simulink model "Type1_c"  (R2019a)
settings: Solver=VariableStepAuto  StartTime=0.0  StopTime=10.0  RelTol=1e-3
libraries: simulink x3
settings Model: Creator=admin  LastModifiedBy=admin

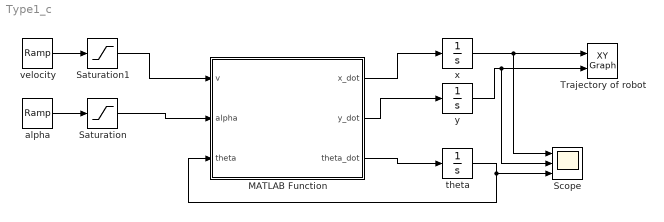
== system Type1_c ==
  MATLAB Function : MATLAB Function  TreatAsAtomicUnit=on
  Saturation : Saturate  UpperLimit=pi/4  LowerLimit=-pi/4
  Saturation1 : Saturate  UpperLimit=1.68  LowerLimit=-1.68  LinearizeAsGain=off
  Scope : Scope  NumInputPorts=3
  Trajectory of robot : simulink/Sinks/XY Graph  xmin=-2  xmax=7  ymin=-1  ymax=5  st=-1
  alpha : simulink/Sources/Ramp  slope=0.6  start=0  InitialOutput=0
  theta : Integrator
  velocity : simulink/Sources/Ramp  slope=0.3  start=0  InitialOutput=0
  x : Integrator
  y : Integrator
  wires:
  x/1 -> Trajectory of robot/1, Scope/1
  theta/1 -> Scope/3, MATLAB Function/3(theta)
  MATLAB Function/2(y_dot) -> y/1
  MATLAB Function/3(theta_dot) -> theta/1
  MATLAB Function/1(x_dot) -> x/1
  y/1 -> Scope/2, Trajectory of robot/2
  Saturation/1 -> MATLAB Function/2(alpha)
  velocity/1 -> Saturation1/1
  Saturation1/1 -> MATLAB Function/1(v)
  alpha/1 -> Saturation/1

== matlab function Type1_c/MATLAB Function ==
  data: v input; x_dot output; alpha input; y_dot output; theta_dot output; theta input
function [x_dot, y_dot, theta_dot] = tricycle_type_1(v, alpha,theta)
d = sqrt(3.1)
x_dot = v*cos(alpha)*cos(theta);
y_dot = v*cos(alpha)*sin(theta);
theta_dot = v/d*sin(alpha);
